simulink model "FutureGridSLs"  (R2024a)
settings: Solver=VariableStepAuto  StartTime=0.0  StopTime=600  FixedStep=1e-3  RelTol=1e-3
values from neighbouring files (symbols this model uses):
  AGG_SOL_R = inf    [FUtureGridSL.m]
  AGG_SOL_S_nom = 980e6    (= 980000000)    [FUtureGridSL.m]
  AGG_SOL_T_INV = 0.02    [FUtureGridSL.m]
  AMB_T_INV = 0.05    [FUtureGridSL.m]
  AMB_Unit_S_nom = 3e6    (= 3000000)    [FUtureGridSL.m]
  BAR_R = 0.04    [FUtureGridSL.m]
  BAR_T_ACT = 0.1    [FUtureGridSL.m]
  BAR_Unit_S_nom = 15e6    (= 15000000)    [FUtureGridSL.m]
  BRO_R_P = 0.05    [FUtureGridSL.m]    (also in Sri_Lanka_FINAL.m)
  BRO_R_T = 0.38    [FUtureGridSL.m]    (also in Sri_Lanka_FINAL.m)
  BRO_T_G = 0.2    [FUtureGridSL.m]    (also in Sri_Lanka_FINAL.m)
  BRO_T_R = 5.0    (= 5)    [FUtureGridSL.m]    (also in Sri_Lanka_FINAL.m)
  BRO_T_W = 1.0    (= 1)    [FUtureGridSL.m]    (also in Sri_Lanka_FINAL.m)
  BRO_Unit_S_nom = 17.5e6    (= 17500000)    [FUtureGridSL.m]    (also in Sri_Lanka_FINAL.m)
  BWT_R_P = 0.05    [FUtureGridSL.m]    (also in Sri_Lanka.m; Sri_Lanka_FINAL.m)
  BWT_R_T = 0.38    [FUtureGridSL.m]    (also in Sri_Lanka.m; Sri_Lanka_FINAL.m)
  BWT_T_R = 5.0    (= 5)    [FUtureGridSL.m]    (also in Sri_Lanka.m; Sri_Lanka_FINAL.m)
  BWT_T_W = 1.5    [FUtureGridSL.m]    (also in Sri_Lanka.m; Sri_Lanka_FINAL.m)
  BWT_Unit_S_nom = 40e6    (= 40000000)    [FUtureGridSL.m]    (also in Sri_Lanka.m; Sri_Lanka_FINAL.m)
  CAN_R_P = 0.05    [FUtureGridSL.m]    (also in Sri_Lanka_FINAL.m)
  CAN_R_T = 0.38    [FUtureGridSL.m]    (also in Sri_Lanka_FINAL.m)
  CAN_T_G = 0.2    [FUtureGridSL.m]    (also in Sri_Lanka_FINAL.m)
  CAN_T_R = 5.0    (= 5)    [FUtureGridSL.m]    (also in Sri_Lanka_FINAL.m)
  CAN_T_W = 1.0    (= 1)    [FUtureGridSL.m]    (also in Sri_Lanka_FINAL.m)
  CAN_Unit_S_nom = 30e6    (= 30000000)    [FUtureGridSL.m]    (also in Sri_Lanka_FINAL.m)
  D_T = 1500e6/S_base_sys    (= 1.5)    [FUtureGridSL.m]    (also in Sri_Lanka.m; Sri_Lanka_FINAL.m)
  f_base = 50    [FUtureGridSL.m]    (also in Sri_Lanka.m; Sri_Lanka_FINAL.m)
  H_eq = sum(Plant_H .* Plant_S_nom .* Plant_Status) / S_base_sys    [FUtureGridSL.m]    (also in Sri_Lanka.m = sum(Plant_H .* Plant_S_nom) / S_base_sys; Sri_Lanka_FINAL.m = sum(Plant_H .* Plant_S_nom) / S_base_sys)
  HBT_S_nom = 1.2e6    (= 1200000)    [FUtureGridSL.m]
  HBT_T_INV = 0.02    [FUtureGridSL.m]
  KEL_CC_F_GT = 0.67    [FUtureGridSL.m]    (also in Sri_Lanka.m; Sri_Lanka_FINAL.m)
  KEL_CC_F_ST = 0.33    [FUtureGridSL.m]    (also in Sri_Lanka.m; Sri_Lanka_FINAL.m)
  KEL_CC_T_HRSG = 10.0    (= 10)    [FUtureGridSL.m]    (also in Sri_Lanka.m; Sri_Lanka_FINAL.m)
  KEL_R = 0.04    [FUtureGridSL.m]    (also in Sri_Lanka.m; Sri_Lanka_FINAL.m)
  KEL_T_CH = 0.3    [FUtureGridSL.m]    (also in Sri_Lanka.m; Sri_Lanka_FINAL.m)
  KEL_UNIT1_S_nom = 20e6    (= 20000000)    [FUtureGridSL.m]    (also in Sri_Lanka.m; Sri_Lanka_FINAL.m)
  KEL_UNIT2_S_nom = 115e6    (= 115000000)    [FUtureGridSL.m]    (also in Sri_Lanka.m; Sri_Lanka_FINAL.m)
  KEL_UNIT3_S_nom = 165e6    (= 165000000)    [FUtureGridSL.m]    (also in Sri_Lanka.m; Sri_Lanka_FINAL.m)
  KOT_R_P = 0.05    [FUtureGridSL.m]
  KOT_R_T = 0.38    [FUtureGridSL.m]
  KOT_T_R = 5.0    (= 5)    [FUtureGridSL.m]
  KOT_T_W = 1.1    [FUtureGridSL.m]
  KOT_Unit_S_nom = 67e6    (= 67000000)    [FUtureGridSL.m]
  KUK_R_P = 0.05    [FUtureGridSL.m]    (also in Sri_Lanka_FINAL.m)
  KUK_R_T = 0.38    [FUtureGridSL.m]    (also in Sri_Lanka_FINAL.m)
  KUK_T_R = 5.0    (= 5)    [FUtureGridSL.m]    (also in Sri_Lanka_FINAL.m)
  KUK_T_W = 0.8    [FUtureGridSL.m]    (also in Sri_Lanka_FINAL.m)
  KUK_Unit_S_nom = 40e6    (= 40000000)    [FUtureGridSL.m]    (also in Sri_Lanka_FINAL.m)
  LAK_R = 0.04    [FUtureGridSL.m]    (also in Sri_Lanka.m; Sri_Lanka_FINAL.m)
  LAK_S_nom = 300e6    (= 300000000)    [FUtureGridSL.m]    (also in Sri_Lanka.m; Sri_Lanka_FINAL.m)
  LAU_T_INV = 0.02    [FUtureGridSL.m]
  LAU_Unit_S_nom = 20e6    (= 20000000)    [FUtureGridSL.m]
  Load_pu = 2388.8 / 1000    (= 2.3888)    [FUtureGridSL.m]
  MAD_T_INV = 0.02    [FUtureGridSL.m]
  MAD_Unit_S_nom = 100e6    (= 100000000)    [FUtureGridSL.m]
  MADK_Unit_S_nom = 12e6    (= 12000000)    [FUtureGridSL.m]
  MADU_T_INV = 0.05    [FUtureGridSL.m]
  MAM1_T_INV = 0.05    [FUtureGridSL.m]
  MAM1_Unit_S_nom = 10e6    (= 10000000)    [FUtureGridSL.m]
  MAM2_T_INV = 0.05    [FUtureGridSL.m]
  MAM2_Unit_S_nom = 10e6    (= 10000000)    [FUtureGridSL.m]
  MAM3_T_INV = 0.05    [FUtureGridSL.m]
  MAM3_Unit_S_nom = 10e6    (= 10000000)    [FUtureGridSL.m]
  MAN_T_INV = 0.05    [FUtureGridSL.m]    (also in Sri_Lanka_FINAL.m)
  MAN_Unit_S_nom = 100e6    (= 100000000)    [FUtureGridSL.m]    (also in Sri_Lanka_FINAL.m)
  NAL_T_INV = 0.05    [FUtureGridSL.m]
  NAL_Unit_S_nom = 4.8e6    (= 4800000)    [FUtureGridSL.m]
  NIR_T_INV = 0.05    [FUtureGridSL.m]
  NIR_Unit_S_nom = 10.5e6    (= 10500000)    [FUtureGridSL.m]
  NLX_R_P = 0.05    [FUtureGridSL.m]    (also in Sri_Lanka_FINAL.m)
  NLX_R_T = 0.40    (= 0.4)    [FUtureGridSL.m]    (also in Sri_Lanka_FINAL.m)
  NLX_T_G = 0.2    [FUtureGridSL.m]    (also in Sri_Lanka_FINAL.m)
  NLX_T_R = 5.0    (= 5)    [FUtureGridSL.m]    (also in Sri_Lanka_FINAL.m)
  NLX_T_W = 1.2    [FUtureGridSL.m]    (also in Sri_Lanka_FINAL.m)
  NLX_Unit_S_nom = 50e6    (= 50000000)    [FUtureGridSL.m]    (also in Sri_Lanka_FINAL.m)
  OLX_R_P = 0.05    [FUtureGridSL.m]    (also in Sri_Lanka_FINAL.m)
  OLX_R_T = 0.38    [FUtureGridSL.m]    (also in Sri_Lanka_FINAL.m)
  OLX_T_G = 0.2    [FUtureGridSL.m]    (also in Sri_Lanka_FINAL.m)
  OLX_T_R = 5.0    (= 5)    [FUtureGridSL.m]    (also in Sri_Lanka_FINAL.m)
  OLX_T_W = 1.0    (= 1)    [FUtureGridSL.m]    (also in Sri_Lanka_FINAL.m)
  OLX_Unit_S_nom_1 = 12.5e6    (= 12500000)    [FUtureGridSL.m]    (also in Sri_Lanka_FINAL.m)
  OLX_Unit_S_nom_2 = 8.33e6    (= 8330000)    [FUtureGridSL.m]    (also in Sri_Lanka_FINAL.m)
  POL_R_P = 0.05    [FUtureGridSL.m]    (also in Sri_Lanka_FINAL.m)
  POL_R_T = 0.40    (= 0.4)    [FUtureGridSL.m]    (also in Sri_Lanka_FINAL.m)
  POL_T_G = 0.2    [FUtureGridSL.m]    (also in Sri_Lanka_FINAL.m)
  POL_T_R = 5.0    (= 5)    [FUtureGridSL.m]    (also in Sri_Lanka_FINAL.m)
  POL_T_W = 1.4    [FUtureGridSL.m]    (also in Sri_Lanka_FINAL.m)
  POL_Unit_S_nom = 45e6    (= 45000000)    [FUtureGridSL.m]    (also in Sri_Lanka_FINAL.m)
  POLW_T_INV = 0.05    [FUtureGridSL.m]
  POLW_Unit_S_nom = 12e6    (= 12000000)    [FUtureGridSL.m]
  Pref_Set_AGG_SOL = (Load_pu * K_AGG_SOL)  * (S_base_sys / AGG_SOL_S_nom)    (= 0)    [FUtureGridSL.m]
  Pref_Set_AMB = (Load_pu * K_AMB) * (S_base_sys / AMB_Unit_S_nom)    (= 0)    [FUtureGridSL.m]
  Pref_Set_BAR = (Load_pu * K_BAR) * (S_base_sys / (4 * BAR_Unit_S_nom))    (= 3.98133333333)    [FUtureGridSL.m]
  Pref_Set_BRO = (Load_pu * K_BRO) * (S_base_sys / (2 * BRO_Unit_S_nom))    (= 0)    [FUtureGridSL.m]
  Pref_Set_BWT = (Load_pu * K_BWT) * (S_base_sys / (1 * BWT_Unit_S_nom))    (= 0)    [FUtureGridSL.m]
  Pref_Set_CAN = (Load_pu * K_CAN) * (S_base_sys / (2 * CAN_Unit_S_nom))    (= 0)    [FUtureGridSL.m]
  Pref_Set_HBT = (Load_pu * K_HBT)  * (S_base_sys / HBT_S_nom)    (= 0)    [FUtureGridSL.m]
  Pref_Set_KEL1 = (Load_pu * K_KEL1)  * (S_base_sys / (4*KEL_UNIT1_S_nom))    (= 0)    [FUtureGridSL.m]
  Pref_Set_KEL2 = (Load_pu * K_KEL2)  * (S_base_sys / (KEL_UNIT2_S_nom ))    (= 0)    [FUtureGridSL.m]
  Pref_Set_KEL3 = (Load_pu * K_KEL3)  * (S_base_sys / (KEL_UNIT3_S_nom))    (= 0)    [FUtureGridSL.m]
  Pref_Set_KOT = (Load_pu * K_KOT)  * (S_base_sys / (3 * KOT_Unit_S_nom))    (= 0.986419900498)    [FUtureGridSL.m]
  Pref_Set_KUK = (Load_pu * K_KUK) * (S_base_sys / (2 * KUK_Unit_S_nom))    (= 0)    [FUtureGridSL.m]
  Pref_Set_LAK = (Load_pu * K_LAK)  * (S_base_sys / (3 * LAK_S_nom))    (= 0.177302044444)    [FUtureGridSL.m]
  Pref_Set_LAU = (Load_pu * K_LAU)  * (S_base_sys / LAU_Unit_S_nom)    (= 1.1944)    [FUtureGridSL.m]
  Pref_Set_MAD = (Load_pu * K_MAD)  * (S_base_sys / MAD_Unit_S_nom)    (= 0.7333616)    [FUtureGridSL.m]
  Pref_Set_MADK = (Load_pu * K_MADK) * (S_base_sys / AMB_Unit_S_nom)    (= 0)    [FUtureGridSL.m]
  Pref_Set_MAM1 = (Load_pu * K_MAM1) * (S_base_sys / MAM1_Unit_S_nom)    (= 0)    [FUtureGridSL.m]
  Pref_Set_MAM2 = (Load_pu * K_MAM2) * (S_base_sys / MAM2_Unit_S_nom)    (= 0)    [FUtureGridSL.m]
  Pref_Set_MAM3 = (Load_pu * K_MAM3) * (S_base_sys / MAM3_Unit_S_nom)    (= 0)    [FUtureGridSL.m]
  Pref_Set_MAN = (Load_pu * K_MAN)  * (S_base_sys / MAN_Unit_S_nom)    (= 0.035832)    [FUtureGridSL.m]
  Pref_Set_NAL = (Load_pu * K_NAL) * (S_base_sys / NAL_Unit_S_nom)    (= 0)    [FUtureGridSL.m]
  Pref_Set_NIR = (Load_pu * K_NIR) * (S_base_sys / NIR_Unit_S_nom)    (= 0)    [FUtureGridSL.m]
  Pref_Set_NLX = (Load_pu * K_NLX)  * (S_base_sys / (2 * NLX_Unit_S_nom))    (= 0)    [FUtureGridSL.m]
  Pref_Set_OLX1 = (Load_pu * K_OLX1) * (S_base_sys / (2 * OLX_Unit_S_nom_1))    (= 0)    [FUtureGridSL.m]
  Pref_Set_OLX2 = (Load_pu * K_OLX2) * (S_base_sys / (3 * OLX_Unit_S_nom_2))    (= 0)    [FUtureGridSL.m]
  Pref_Set_POL = (Load_pu * K_POL) * (S_base_sys / (2 * POL_Unit_S_nom))    (= 0)    [FUtureGridSL.m]
  Pref_Set_POLW = (Load_pu * K_POLW) * (S_base_sys / POLW_Unit_S_nom)    (= 0)    [FUtureGridSL.m]
  Pref_Set_PWD = (Load_pu * K_PWD) * (S_base_sys / PWD_Unit_S_nom)    (= 0)    [FUtureGridSL.m]
  Pref_Set_RAN = (Load_pu * K_RAN) * (S_base_sys / (2 * RAN_Unit_S_nom))    (= 9.47936507937)    [FUtureGridSL.m]
  Pref_Set_RTB = (Load_pu * K_RTB) * (S_base_sys / (2 * RTB_Unit_S_nom))    (= 0)    [FUtureGridSL.m]
  ... (+116 more)
(part 2 of 2)

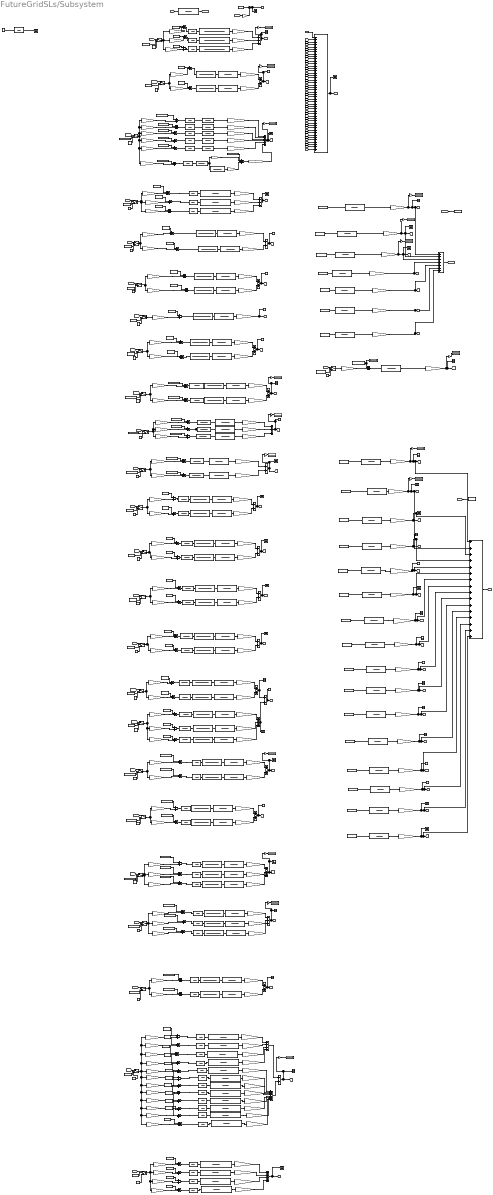
== system FutureGridSLs/Subsystem ==
  note: HambanthotaSolarFarm
  note: [Steam Turbine Path: 33%]
  note: [Gas Turbine Path: 67%]
  note: SAMANALAWEWA
  note: GRID BLOCK
  note: SUMMING BLOCK
  note: To convert to the frequency
  note: LAKVIJAYA
  note: KELANITISSA
  note: Uthuru Janani plant
  note: RANDENIGALA
  note: RANTAMBE
  note: BOWATENNA
  note: UKUWELA
  note: Yugadhanavi GT and ST
  note: New LAXAPANA
  note: Sobadhanavi ST and GT
  note: Polpitiya Plant
  note: Canyon Plant
  note: Wimalasurendra Plant
  note: Kukuleganga Plant
  note: Uma Oya Plant
  note: Old Laxapana Plant
  note: Broadland Plant
  note: Victoria Plant
  note: Upper Kotmale Plant
  note: Kotmale Plant
  note: Colombo Port Barge Plant
  note: Sapugaskanda Plant
  note: Uppudaluwa Wind Farm
  note: Maduru Oya Solar PV subsystem
  note: LAUGFS Hambantota Solar Power Plant
  note: Solar One Ceylon Solar Farm
  note: THAMBAPAVANI WIND FARM: 100 MW
  note: SagaSolarFarm
  note: Suryashakthi 1 SolarFarm
  note: Suryashakthi 2 SolarFarm
  note: Ambewela Aitken Spence Wind Farm
  note: Madurankuliya Wind Farm
  note: Mampuri I Wind Farm
  note: Mampuri II Wind Farm
  note: Mampuri III Wind Farm
  note: Nala Danavi Wind Farm
  note: Nirmalapura Wind Farm
  note: Pawan Danavi Wind Farm
  note: Pollupalai Wind Farm
  note: Seguwantivu Wind Farm
  note: Vallimunai Wind Farm
  note: Vidatamunai Wind Farm
  note: Willwind Wind Farm
  note: Wind scape Farm
  note: Forecasted Solar PV Farm (IBR)
  Load Disturbance : Inport
  " " : TransferFcn  Denominator=[2*H_eq D_T]
  Actuator Delay : TransferFcn  Denominator="[UTH_T_ACT  1]"
  Actuator Delay1 : TransferFcn  Denominator="[UTH_T_ACT  1]"
  Actuator Delay{3..13,15} (12 alike) : TransferFcn  Denominator="[SAP_T_ACT  1]"
  Actuator Delay{14,16..18} (4 alike) : TransferFcn  Denominator="[BAR_T_ACT  1]"
  Actuator Delay2 : TransferFcn  Denominator="[UTH_T_ACT  1]"
  Add{,4,8,13,20..21} (6 alike) : Sum  Inputs=+++
  Add1 : Sum  Inputs=-+++++++++++++++++++++++++++++++++++++++++++++++
  Add{2,5..7,9..12,14..19,22,25,27,29..65,67..98} (86 alike) : Sum
  Add23 : Sum  Inputs=++++
  Add24 : Sum  Inputs=++++++++
  Add26 : Sum  Inputs=++++
  Add28 : Sum  Inputs=+++++++
  Add3 : Sum  Inputs=++++++
  Add66 : Sum  Inputs=++++++++++++++++
  Base Scaling Gain : Gain  Gain=SAM_Unit_S_nom / S_base_sys
  Base Scaling Gain GT : Gain  Gain=YUGA_GT_S_nom / S_base_sys
  Base Scaling Gain GT1 : Gain  Gain=YUGA_GT_S_nom / S_base_sys
  Base Scaling Gain GT2 : Gain  Gain=SOBA_GT_S_nom / S_base_sys
  Base Scaling Gain1 : Gain  Gain=SAM_Unit_S_nom / S_base_sys
  Base Scaling Gain10 : Gain  Gain=RTB_Unit_S_nom / S_base_sys
  Base Scaling Gain11 : Gain  Gain=UKU_Unit_S_nom / S_base_sys
  Base Scaling Gain12 : Gain  Gain=BWT_Unit_S_nom / S_base_sys
  Base Scaling Gain13 : Gain  Gain=UKU_Unit_S_nom / S_base_sys
  Base Scaling Gain14 : Gain  Gain=MAN_Unit_S_nom / S_base_sys
  Base Scaling Gain15 : Gain  Gain=SOBA_ST_S_nom/S_base_sys
  Base Scaling Gain16 : Gain  Gain=YUGA_ST_S_nom/S_base_sys
  Base Scaling Gain17 : Gain  Gain=NLX_Unit_S_nom / S_base_sys
  Base Scaling Gain18 : Gain  Gain=NLX_Unit_S_nom / S_base_sys
  Base Scaling Gain19 : Gain  Gain=POL_Unit_S_nom / S_base_sys
  Base Scaling Gain2 : Gain  Gain=RTB_Unit_S_nom / S_base_sys
  Base Scaling Gain20 : Gain  Gain=POL_Unit_S_nom / S_base_sys
  Base Scaling Gain21 : Gain  Gain=WIM_Unit_S_nom / S_base_sys
  Base Scaling Gain22 : Gain  Gain=WIM_Unit_S_nom / S_base_sys
  Base Scaling Gain23 : Gain  Gain=BRO_Unit_S_nom / S_base_sys
  Base Scaling Gain24 : Gain  Gain=BRO_Unit_S_nom / S_base_sys
  Base Scaling Gain25 : Gain  Gain=OLX_Unit_S_nom_1 / S_base_sys
  Base Scaling Gain26 : Gain  Gain=OLX_Unit_S_nom_1 / S_base_sys
  Base Scaling Gain27 : Gain  Gain=OLX_Unit_S_nom_2 / S_base_sys
  Base Scaling Gain28 : Gain  Gain=OLX_Unit_S_nom_2 / S_base_sys
  Base Scaling Gain29 : Gain  Gain=OLX_Unit_S_nom_2 / S_base_sys
  Base Scaling Gain{3..6} (4 alike) : Gain  Gain=KEL_UNIT1_S_nom/ S_base_sys
  Base Scaling Gain30 : Gain  Gain=UMA_Unit_S_nom / S_base_sys
  Base Scaling Gain31 : Gain  Gain=UMA_Unit_S_nom / S_base_sys
  Base Scaling Gain32 : Gain  Gain=KUK_Unit_S_nom / S_base_sys
  Base Scaling Gain33 : Gain  Gain=KUK_Unit_S_nom / S_base_sys
  Base Scaling Gain34 : Gain  Gain=CAN_Unit_S_nom / S_base_sys
  Base Scaling Gain35 : Gain  Gain=CAN_Unit_S_nom / S_base_sys
  Base Scaling Gain36 : Gain  Gain=VIC_Unit_S_nom / S_base_sys
  Base Scaling Gain37 : Gain  Gain=VIC_Unit_S_nom / S_base_sys
  Base Scaling Gain38 : Gain  Gain=VIC_Unit_S_nom / S_base_sys
  Base Scaling Gain39 : Gain  Gain=KOT_Unit_S_nom / S_base_sys
  Base Scaling Gain40 : Gain  Gain=KOT_Unit_S_nom / S_base_sys
  Base Scaling Gain41 : Gain  Gain=UKT_Unit_S_nom / S_base_sys
  Base Scaling Gain42 : Gain  Gain=UKT_Unit_S_nom / S_base_sys
  Base Scaling Gain43 : Gain  Gain=KOT_Unit_S_nom / S_base_sys
  Base Scaling Gain44 : Gain  Gain=MAD_Unit_S_nom / S_base_sys
  Base Scaling Gain45 : Gain  Gain=LAU_Unit_S_nom / S_base_sys
  Base Scaling Gain46 : Gain  Gain=SOC_S_nom / S_base_sys
  Base Scaling Gain47 : Gain  Gain=UPP_Unit_S_nom / S_base_sys
  Base Scaling Gain49 : Gain  Gain=HBT_S_nom / S_base_sys
  Base Scaling Gain50 : Gain  Gain=SAG_S_nom / S_base_sys
  Base Scaling Gain51 : Gain  Gain=SS1_S_nom / S_base_sys
  Base Scaling Gain52 : Gain  Gain=SS2_S_nom / S_base_sys
  Base Scaling Gain53 : Gain  Gain=AMB_Unit_S_nom / S_base_sys
  Base Scaling Gain54 : Gain  Gain=MADK_Unit_S_nom / S_base_sys
  Base Scaling Gain55 : Gain  Gain=MAM1_Unit_S_nom / S_base_sys
  Base Scaling Gain56 : Gain  Gain=MAM2_Unit_S_nom / S_base_sys
  Base Scaling Gain57 : Gain  Gain=MAM3_Unit_S_nom / S_base_sys
  Base Scaling Gain58 : Gain  Gain=NAL_Unit_S_nom / S_base_sys
  Base Scaling Gain59 : Gain  Gain=NIR_Unit_S_nom / S_base_sys
  Base Scaling Gain60 : Gain  Gain=PWD_Unit_S_nom / S_base_sys
  Base Scaling Gain61 : Gain  Gain=POLW_Unit_S_nom / S_base_sys
  Base Scaling Gain62 : Gain  Gain=SEG_Unit_S_nom / S_base_sys
  Base Scaling Gain63 : Gain  Gain=AGG_SOL_S_nom / S_base_sys
  Base Scaling Gain64 : Gain  Gain=VALL_Unit_S_nom / S_base_sys
  Base Scaling Gain65 : Gain  Gain=VID_Unit_S_nom / S_base_sys
  Base Scaling Gain66 : Gain  Gain=WILL_Unit_S_nom / S_base_sys
  Base Scaling Gain67 : Gain  Gain=WSC_Unit_S_nom / S_base_sys
  Base Scaling Gain7 : Gain  Gain=KEL_UNIT2_S_nom/ S_base_sys
  Base Scaling Gain8 : Gain  Gain=RAN_Unit_S_nom / S_base_sys
  Base Scaling Gain9 : Gain  Gain=RAN_Unit_S_nom / S_base_sys
  Combustr : TransferFcn  Denominator="[KEL_T_CH  1]"
  Constant : Constant  Value=f_base
  Constant{1,15..16,143} (4 alike) : Constant  Value=Pref_Set_LAK
  Constant10 : Constant  Value=Pref_Set_MAN
  Constant{22,96..118,127,144} (26 alike) : Constant  Value=0
  Constant11 : Constant  Value=Pref_Set_MAD
  Constant{92..95,119} (5 alike) : Constant  Value=Pref_Set_BAR
  Constant12 : Constant  Value=Pref_Set_LAU
  Constant{33..36,120} (5 alike) : Constant  Value=Pref_Set_SAP_A
  Constant121 : Constant  Value=Pref_Set_UKT
  Constant{30..32,122} (4 alike) : Constant  Value=Pref_Set_KOT
  Constant{27..29,123} (4 alike) : Constant  Value=Pref_Set_VIC
  Constant124 : Constant  Value=Pref_Set_KUK
  Constant125 : Constant  Value=Pref_Set_UMA
  Constant126 : Constant  Value=Pref_Set_OLX1
  Constant{85..87,128} (4 alike) : Constant  Value=Pref_Set_OLX2
  Constant129 : Constant  Value=Pref_Set_BRO
  Constant13 : Constant  Value=Pref_Set_SOC
  Constant130 : Constant  Value=Pref_Set_WIM
  Constant131 : Constant  Value=Pref_Set_CAN
  Constant132 : Constant  Value=Pref_Set_POL
  Constant133 : Constant  Value=Pref_Set_SOBA1
  Constant134 : Constant  Value=Pref_Set_YUGA1
  Constant135 : Constant  Value=Pref_Set_NLX
  Constant136 : Constant  Value=Pref_Set_UKU
  Constant137 : Constant  Value=Pref_Set_BWT
  Constant138 : Constant  Value=Pref_Set_RTB
  Constant139 : Constant  Value=Pref_Set_RAN
  Constant14 : Constant  Value=Pref_Set_UPP
  Constant{61,66..67,140} (4 alike) : Constant  Value=Pref_Set_UTH
  Constant{5,18..20,141} (5 alike) : Constant  Value=Pref_Set_KEL1
  Constant142 : Constant  Value=Pref_Set_SAM
  Constant145 : Constant  Value=Pref_Set_AGG_SOL
  Constant146 : Constant  Value=Pref_Set_AGG_SOL
  Constant17 : Constant  Value=Pref_Set_SAM
  Constant2 : Constant
  Constant21 : Constant  Value=Pref_Set_KEL2
  Constant23 : Constant  Value=Pref_Set_NLX
  Constant24 : Constant  Value=Pref_Set_NLX
  Constant25 : Constant  Value=Pref_Set_UMA
  Constant26 : Constant  Value=Pref_Set_UMA
  Constant{37..44} (8 alike) : Constant  Value=Pref_Set_SAP_B
  Constant4 : Constant  Value=Pref_Set_SAM
  Constant45 : Constant  Value=Pref_Set_SOBA1
  Constant46 : Constant  Value=Pref_Set_SOBA2
  Constant47 : Constant  Value=Pref_Set_HBT
  Constant48 : Constant  Value=Pref_Set_SAG
  Constant49 : Constant  Value=Pref_Set_SS1
  Constant50 : Constant  Value=Pref_Set_SS2
  Constant51 : Constant  Value=Pref_Set_AMB
  Constant52 : Constant  Value=Pref_Set_MADK
  Constant53 : Constant  Value=Pref_Set_MAM1
  Constant54 : Constant  Value=Pref_Set_MAM2
  Constant55 : Constant  Value=Pref_Set_MAM3
  Constant56 : Constant  Value=Pref_Set_NAL
  Constant57 : Constant  Value=Pref_Set_NIR
  Constant58 : Constant  Value=Pref_Set_PWD
  Constant59 : Constant  Value=Pref_Set_POLW
  Constant6 : Constant  Value=Pref_Set_YUGA1
  Constant60 : Constant  Value=Pref_Set_SEG
  Constant62 : Constant  Value=Pref_Set_VALL
  Constant63 : Constant  Value=Pref_Set_VID
  Constant64 : Constant  Value=Pref_Set_WILL
  Constant65 : Constant  Value=Pref_Set_WSC
  Constant68 : Constant  Value=Pref_Set_RAN
  Constant69 : Constant  Value=Pref_Set_RAN
  Constant7 : Constant  Value=Pref_Set_YUGA1
  Constant70 : Constant  Value=Pref_Set_RTB
  Constant71 : Constant  Value=Pref_Set_RTB
  Constant72 : Constant  Value=Pref_Set_BWT
  Constant73 : Constant  Value=Pref_Set_UKU
  Constant74 : Constant  Value=Pref_Set_UKU
  Constant75 : Constant  Value=Pref_Set_POL
  Constant76 : Constant  Value=Pref_Set_POL
  Constant77 : Constant  Value=Pref_Set_CAN
  Constant78 : Constant  Value=Pref_Set_CAN
  Constant79 : Constant  Value=Pref_Set_WIM
  Constant8 : Constant  Value=Pref_Set_YUGA2
  Constant80 : Constant  Value=Pref_Set_WIM
  Constant81 : Constant  Value=Pref_Set_BRO
  Constant82 : Constant  Value=Pref_Set_BRO
  Constant83 : Constant  Value=Pref_Set_OLX1
  Constant84 : Constant  Value=Pref_Set_OLX1
  Constant88 : Constant  Value=Pref_Set_KUK
  Constant89 : Constant  Value=Pref_Set_KUK
  Constant9 : Constant  Value=Pref_Set_KEL3
  Constant90 : Constant  Value=Pref_Set_UKT
  Constant91 : Constant  Value=Pref_Set_UKT
  Display{,1..16} (17 alike) : Display
  Gain{,4..8,13..18} (12 alike) : Gain  Gain=1e3
  Gain1 : Gain  Gain=KEL_CC_F_ST
  Gain10 : Gain  Gain=(3*VIC_Unit_S_nom)/ 1e6
  Gain11 : Gain  Gain=(3*KOT_Unit_S_nom)/ 1e6
  Gain12 : Gain  Gain=(4*SAP_A_Unit_S_nom + 8*SAP_B_Unit_S_nom)/1e6
  Gain2 : Gain  Gain=KEL_UNIT3_S_nom/ S_base_sys
  Gain3 : Gain  Gain=f_base
  Gain9 : Gain  Gain=(2*UMA_Unit_S_nom)/ 1e6
  Governer{,1..13} (14 alike) : TransferFcn  Denominator=[T_G 1]
  Governer {1..2,7,9,11,13,15,17..19,30..33,35..46} (26 alike) : TransferFcn  Denominator=[T_G 1]
  Governer {8,10,12,14,16} (5 alike) : TransferFcn  Denominator="[KEL_T_CH  1]"
  Governer 20 : TransferFcn  Denominator=[CAN_T_G 1]
  Governer 21 : TransferFcn  Denominator="[WIM_T_G  1]"
  Governer 22 : TransferFcn  Denominator="[WIM_T_G  1]"
  Governer 23 : TransferFcn  Denominator="[BRO_T_G  1]"
  Governer 24 : TransferFcn  Denominator="[BRO_T_G  1]"
  Governer {25..29} (5 alike) : TransferFcn  Denominator="[OLX_T_G  1]"
  Governer 3 : TransferFcn  Denominator=[POL_T_G 1]
  Governer 34 : TransferFcn  Denominator="[CAN_T_G  1]"
  Governer 4 : TransferFcn  Denominator=[POL_T_G 1]
  Governer 47 : TransferFcn  Denominator=[100 1]
  Governer 5 : TransferFcn  Denominator=[NLX_T_G 1]
  Governer 6 : TransferFcn  Denominator=[NLX_T_G 1]
  Governer GT : TransferFcn  Denominator=[YUGA_GT_T_G 1]
  Governer GT1 : TransferFcn  Denominator=[YUGA_GT_T_G 1]
  Governer GT2 : TransferFcn  Denominator=[SOBA_GT_T_g 1]
  Governer ST : TransferFcn  Denominator=[YUGA_ST_T_ch 1]
  Governer ST1 : TransferFcn  Denominator=[SOBA_ST_T_ch 1]
  HRSG Delay : TransferFcn  Denominator="[KEL_CC_T_HRSG  1]"
  Inverter Delay : TransferFcn  Denominator="[MAN_T_INV  1]"
  Inverter Delay1 : TransferFcn  Denominator=[MAD_T_INV 1]
  Inverter Delay10 : TransferFcn  Denominator=[MADU_T_INV 1]
  Inverter Delay11 : TransferFcn  Denominator=[MAM1_T_INV 1]
  Inverter Delay12 : TransferFcn  Denominator=[MAM2_T_INV 1]
  Inverter Delay13 : TransferFcn  Denominator=[MAM3_T_INV 1]
  Inverter Delay14 : TransferFcn  Denominator=[NAL_T_INV 1]
  Inverter Delay15 : TransferFcn  Denominator=[NIR_T_INV 1]
  Inverter Delay16 : TransferFcn  Denominator=[PWD_T_INV 1]
  Inverter Delay17 : TransferFcn  Denominator=[POLW_T_INV 1]
  Inverter Delay18 : TransferFcn  Denominator=[SEG_T_INV 1]
  Inverter Delay2 : TransferFcn  Denominator=[LAU_T_INV 1]
  Inverter Delay20 : TransferFcn  Denominator=[VALL_T_INV 1]
  Inverter Delay21 : TransferFcn  Denominator=[VID_T_INV 1]
  Inverter Delay22 : TransferFcn  Denominator=[WILL_T_INV 1]
  Inverter Delay23 : TransferFcn  Denominator=[WSC_T_INV 1]
  Inverter Delay3 : TransferFcn  Denominator=[SOC_T_INV 1]
  Inverter Delay4 : TransferFcn  Denominator=[UPP_T_INV 1]
  Inverter Delay5 : TransferFcn  Denominator=[HBT_T_INV 1]
  Inverter Delay6 : TransferFcn  Denominator=[SAG_T_INV 1]
  Inverter Delay7 : TransferFcn  Denominator=[SS1_T_INV 1]
  Inverter Delay8 : TransferFcn  Denominator=[SS2_T_INV 1]
  Inverter Delay9 : TransferFcn  Denominator=[AMB_T_INV 1]
  PURE DROOP : Gain  Gain=-1/LAK_R
  PURE DROOP GT : Gain  Gain=-1/YUGA_GT_R
  PURE DROOP GT1 : Gain  Gain=-1/YUGA_GT_R
  PURE DROOP GT2 : Gain  Gain=-1/SOBA_GT_R
  PURE DROOP ST : Gain  Gain=-1/YUGA_ST_R
  PURE DROOP ST1 : Gain  Gain=-1/SOBA_ST_R
  PURE DROOP1 : Gain  Gain=-1/LAK_R
  PURE DROOP{6..11} (6 alike) : Gain  Gain=-1/KEL_R
  PURE DROOP12 : Gain  Gain=-1/UTH_R
  PURE DROOP13 : Gain  Gain=-1/UTH_R
  PURE DROOP14 : Gain  Gain=-1/UTH_R
  PURE DROOP15 : Gain  Gain=-1/RAN_R_P
  PURE DROOP16 : Gain  Gain=-1/RAN_R_P
  PURE DROOP17 : Gain  Gain=-1/RTB_R_P
  PURE DROOP18 : Gain  Gain=-1/UKU_R_P
  PURE DROOP19 : Gain  Gain=-1/BWT_R_P
  PURE DROOP2 : Gain  Gain=-1/LAK_R
  PURE DROOP20 : Gain  Gain=-1/UKU_R_P
  PURE DROOP21 : Gain  Gain=-1/AGG_SOL_R
  PURE DROOP22 : Gain  Gain=-1/NLX_R_P
  PURE DROOP23 : Gain  Gain=-1/NLX_R_P
  PURE DROOP24 : Gain  Gain=-1/POL_R_P
  PURE DROOP25 : Gain  Gain=-1/POL_R_P
  PURE DROOP26 : Gain  Gain=-1/CAN_R_P
  PURE DROOP27 : Gain  Gain=-1/WIM_R_P
  PURE DROOP28 : Gain  Gain=-1/WIM_R_P
  PURE DROOP29 : Gain  Gain=-1/BRO_R_P
  PURE DROOP3 : Gain  Gain=-1/SAM_R_P
  PURE DROOP30 : Gain  Gain=-1/BRO_R_P
  PURE DROOP{31..35} (5 alike) : Gain  Gain=-1/OLX_R_P
  PURE DROOP36 : Gain  Gain=-1/UMA_R_P
  PURE DROOP37 : Gain  Gain=-1/UMA_R_P
  PURE DROOP38 : Gain  Gain=-1/KUK_R_P
  PURE DROOP39 : Gain  Gain=-1/KUK_R_P
  PURE DROOP4 : Gain  Gain=-1/SAM_R_P
  PURE DROOP40 : Gain  Gain=-1/CAN_R_P
  PURE DROOP41 : Gain  Gain=-1/VIC_R_P
  PURE DROOP42 : Gain  Gain=-1/VIC_R_P
  PURE DROOP43 : Gain  Gain=-1/VIC_R_P
  PURE DROOP44 : Gain  Gain=-1/KOT_R_P
  PURE DROOP45 : Gain  Gain=-1/KOT_R_P
  PURE DROOP46 : Gain  Gain=-1/UKT_R_P
  PURE DROOP47 : Gain  Gain=-1/UKT_R_P
  PURE DROOP48 : Gain  Gain=-1/KOT_R_P
  PURE DROOP{49..60} (12 alike) : Gain  Gain=-1/SAP_R
  PURE DROOP5 : Gain  Gain=-1/RTB_R_P
  PURE DROOP{61..64} (4 alike) : Gain  Gain=-1/BAR_R
  Scaling : Sum  Inputs=+++
  Scaling 1 : Gain  Gain=LAK_S_nom / S_base_sys
  Scaling {7..10} (4 alike) : Gain  Gain=SAP_A_Unit_S_nom / S_base_sys
  Scaling {11..18} (8 alike) : Gain  Gain=SAP_B_Unit_S_nom / S_base_sys
  Scaling {19..22} (4 alike) : Gain  Gain=BAR_Unit_S_nom / S_base_sys
  Scaling 2 : Gain  Gain=LAK_S_nom / S_base_sys
  Scaling 3 : Gain  Gain=LAK_S_nom / S_base_sys
  Scaling 4 : Gain  Gain=UTH_Unit_S_nom / S_base_sys
  Scaling 5 : Gain  Gain=UTH_Unit_S_nom / S_base_sys
  Scaling 6 : Gain  Gain=UTH_Unit_S_nom / S_base_sys
  Scope{,1..31,33..47} (47 alike) : Scope
  Scope32 : Scope  NumInputPorts=2
  Sum : Sum  Inputs=|++
  "Switch " : Switch  Criteria=u2 > Threshold  SaturateOnIntegerOverflow=off  InputSameDT=off
  Switch{1..24} (24 alike) : Switch  Criteria=u2 > Threshold  SaturateOnIntegerOverflow=off  InputSameDT=off
  To Workspace : ToWorkspace  VariableName=SOLAR_TOT  SaveFormat=Timeseries  SampleTime=-1
  To Workspace1 : ToWorkspace  VariableName=WIND_TOT  SaveFormat=Timeseries  SampleTime=-1
  Transient Droop : TransferFcn  Numerator="[SAM_T_R  1]"  Denominator="[SAM_T_R*(SAM_R_T/SAM_R_P)  1]"
  Transient Droop GT : TransferFcn  Denominator="[YUGA_GT_T_t  1]"
  Transient Droop GT1 : TransferFcn  Denominator="[YUGA_GT_T_t  1]"
  Transient Droop GT2 : TransferFcn  Denominator="[SOBA_GT_T_t  1]"
  Transient Droop ST : TransferFcn  Denominator="[YUGA_ST_T_hrsga  1]"
  Transient Droop ST1 : TransferFcn  Denominator="[SOBA_ST_T_hrsga  1]"
  Transient Droop1 : TransferFcn  Numerator="[SAM_T_R  1]"  Denominator="[SAM_T_R*(SAM_R_T/SAM_R_P)  1]"
  Transient Droop10 : TransferFcn  Numerator="[NLX_T_R  1]"  Denominator="[NLX_T_R*(NLX_R_T/NLX_R_P)  1]"
  Transient Droop11 : TransferFcn  Numerator=[POL_T_R 1]  Denominator="[POL_T_R*(POL_R_T/POL_R_P)  1]"
  Transient Droop12 : TransferFcn  Numerator="[POL_T_R  1]"  Denominator="[POL_T_R*(POL_R_T/POL_R_P)  1]"
  Transient Droop13 : TransferFcn  Numerator=[BRO_T_R 1]  Denominator="[BRO_T_R*(BRO_R_T/BRO_R_P)  1]"
  Transient Droop14 : TransferFcn  Numerator=[BRO_T_R 1]  Denominator="[BRO_T_R*(BRO_R_T/BRO_R_P)  1]"
  Transient Droop{15..19} (5 alike) : TransferFcn  Numerator=[OLX_T_R 1]  Denominator="[OLX_T_R*(OLX_R_T/OLX_R_P)  1]"
  Transient Droop2 : TransferFcn  Numerator="[RAN_T_R  1]"  Denominator="[(RAN_R_T / RAN_R_P) * RAN_T_R   1]"
  Transient Droop20 : TransferFcn  Numerator="[UMA_T_R  1]"  Denominator="[UMA_T_R*(UMA_R_T/UMA_R_P)  1]"
  Transient Droop21 : TransferFcn  Numerator="[UMA_T_R  1]"  Denominator="[UMA_T_R*(UMA_R_T/UMA_R_P)  1]"
  Transient Droop22 : TransferFcn  Numerator="[KUK_T_R  1]"  Denominator="[KUK_T_R*(KUK_R_T/KUK_R_P)  1]"
  Transient Droop23 : TransferFcn  Numerator="[KUK_T_R  1]"  Denominator="[KUK_T_R*(KUK_R_T/KUK_R_P)  1]"
  Transient Droop24 : TransferFcn  Numerator=[CAN_T_R 1]  Denominator="[CAN_T_R*(CAN_R_T/CAN_R_P)  1]"
  Transient Droop25 : TransferFcn  Numerator=[CAN_T_R 1]  Denominator="[CAN_T_R*(CAN_R_T/CAN_R_P)  1]"
  Transient Droop26 : TransferFcn  Numerator=[WIM_T_R 1]  Denominator="[WIM_T_R*(WIM_R_T/WIM_R_P)  1]"
  Transient Droop27 : TransferFcn  Numerator=[WIM_T_R 1]  Denominator="[WIM_T_R*(WIM_R_T/WIM_R_P)  1]"
  Transient Droop28 : TransferFcn  Numerator="[VIC_T_R  1]"  Denominator="[VIC_T_R*(VIC_R_T/VIC_R_P)  1]"
  Transient Droop29 : TransferFcn  Numerator="[VIC_T_R  1]"  Denominator="[VIC_T_R*(VIC_R_T/VIC_R_P)  1]"
  Transient Droop3 : TransferFcn  Numerator="[RAN_T_R  1]"  Denominator="[(RAN_R_T / RAN_R_P) * RAN_T_R   1]"
  Transient Droop30 : TransferFcn  Numerator="[VIC_T_R  1]"  Denominator="[VIC_T_R*(VIC_R_T/VIC_R_P)  1]"
  Transient Droop31 : TransferFcn  Numerator="[KOT_T_R  1]"  Denominator="[KOT_T_R*(KOT_R_T/KOT_R_P)  1]"
  Transient Droop32 : TransferFcn  Numerator="[KOT_T_R  1]"  Denominator="[KOT_T_R*(KOT_R_T/KOT_R_P)  1]"
  Transient Droop33 : TransferFcn  Numerator="[UKT_T_R  1]"  Denominator="[UKT_T_R*(UKT_R_T/UKT_R_P)  1]"
  Transient Droop34 : TransferFcn  Numerator="[UKT_T_R  1]"  Denominator="[UKT_T_R*(UKT_R_T/UKT_R_P)  1]"
  Transient Droop35 : TransferFcn  Numerator="[KOT_T_R  1]"  Denominator="[KOT_T_R*(KOT_R_T/KOT_R_P)  1]"
  Transient Droop37 : TransferFcn  Denominator=[AGG_SOL_T_INV, 1]
  Transient Droop4 : TransferFcn  Numerator="[RTB_T_R  1]"  Denominator="[(RTB_R_T / RTB_R_P) * RTB_T_R   1]"
  Transient Droop5 : TransferFcn  Numerator="[RTB_T_R  1]"  Denominator="[(RTB_R_T / RTB_R_P) * RTB_T_R   1]"
  Transient Droop6 : TransferFcn  Numerator="[BWT_T_R  1]"  Denominator="[(BWT_R_T / BWT_R_P) * BWT_T_R   1]"
  Transient Droop7 : TransferFcn  Numerator="[UKU_T_R  1]"  Denominator="[(UKU_R_T / UKU_R_P) * UKU_T_R   1]"
  Transient Droop8 : TransferFcn  Numerator="[UKU_T_R  1]"  Denominator="[(UKU_R_T / UKU_R_P) * UKU_T_R   1]"
  Transient Droop9 : TransferFcn  Numerator=[NLX_T_R 1]  Denominator="[NLX_T_R*(NLX_R_T/NLX_R_P)  1]"
  Turbine Dynamics (Reheat) : TransferFcn  Numerator="[RHT_F_HP*RHT_T_RH  1]"  Denominator="[RHT_T_CH*RHT_T_RH  (RHT_T_CH+RHT_T_RH)  1]"
  Turbine Dynamics (Reheat)1 : TransferFcn  Numerator="[RHT_F_HP*RHT_T_RH  1]"  Denominator="[RHT_T_CH*RHT_T_RH  (RHT_T_CH+RHT_T_RH)  1]"
  Turbine Dynamics (Reheat)2 : TransferFcn  Numerator="[RHT_F_HP*RHT_T_RH  1]"  Denominator="[RHT_T_CH*RHT_T_RH  (RHT_T_CH+RHT_T_RH)  1]"
  Water Column : TransferFcn  Numerator="[-SAM_T_W  1]"  Denominator="[0.5*SAM_T_W  1]"
  Water Column1 : TransferFcn  Numerator="[-SAM_T_W  1]"  Denominator="[0.5*SAM_T_W  1]"
  Water Column10 : TransferFcn  Numerator="[-NLX_T_W  1]"  Denominator="[0.5*NLX_T_W  1]"
  Water Column11 : TransferFcn  Numerator="[-POL_T_W  1]"  Denominator="[0.5*POL_T_W  1]"
  Water Column12 : TransferFcn  Numerator="[-POL_T_W  1]"  Denominator="[0.5*POL_T_W  1]"
  Water Column13 : TransferFcn  Numerator="[-BRO_T_W  1]"  Denominator="[0.5*BRO_T_W  1]"
  Water Column14 : TransferFcn  Numerator="[-BRO_T_W  1]"  Denominator="[0.5*BRO_T_W  1]"
  Water Column{15..19} (5 alike) : TransferFcn  Numerator="[-OLX_T_W  1]"  Denominator="[0.5*OLX_T_W  1]"
  Water Column2 : TransferFcn  Numerator="[-RAN_T_W  1]"  Denominator="[0.5 * RAN_T_W   1]"
  Water Column20 : TransferFcn  Numerator="[-UMA_T_W  1]"  Denominator="[0.5*UMA_T_W  1]"
  Water Column21 : TransferFcn  Numerator="[-UMA_T_W  1]"  Denominator="[0.5*UMA_T_W  1]"
  Water Column22 : TransferFcn  Numerator="[-KUK_T_W  1]"  Denominator="[0.5*KUK_T_W  1]"
  Water Column23 : TransferFcn  Numerator="[-KUK_T_W  1]"  Denominator="[0.5*KUK_T_W  1]"
  Water Column24 : TransferFcn  Numerator="[-CAN_T_W  1]"  Denominator="[0.5*CAN_T_W  1]"
  Water Column25 : TransferFcn  Numerator="[-CAN_T_W  1]"  Denominator="[0.5*CAN_T_W  1]"
  Water Column26 : TransferFcn  Numerator="[-WIM_T_W  1]"  Denominator="[0.5*WIM_T_W  1]"
  Water Column27 : TransferFcn  Numerator="[-WIM_T_W  1]"  Denominator="[0.5*WIM_T_W  1]"
  Water Column28 : TransferFcn  Numerator="[-VIC_T_W  1]"  Denominator="[0.5*VIC_T_W  1]"
  Water Column29 : TransferFcn  Numerator="[-VIC_T_W  1]"  Denominator="[0.5*VIC_T_W  1]"
  Water Column3 : TransferFcn  Numerator="[-RAN_T_W  1]"  Denominator="[0.5 * RAN_T_W   1]"
  Water Column30 : TransferFcn  Numerator="[-VIC_T_W  1]"  Denominator="[0.5*VIC_T_W  1]"
  Water Column31 : TransferFcn  Numerator="[-KOT_T_W  1]"  Denominator="[0.5*KOT_T_W  1]"
  Water Column32 : TransferFcn  Numerator="[-KOT_T_W  1]"  Denominator="[0.5*KOT_T_W  1]"
  Water Column33 : TransferFcn  Numerator="[-UKT_T_W  1]"  Denominator="[0.5*UKT_T_W  1]"
  Water Column34 : TransferFcn  Numerator="[-UKT_T_W  1]"  Denominator="[0.5*UKT_T_W  1]"
  Water Column35 : TransferFcn  Numerator="[-KOT_T_W  1]"  Denominator="[0.5*KOT_T_W  1]"
  Water Column4 : TransferFcn  Numerator="[-RTB_T_W  1]"  Denominator="[0.5 * RTB_T_W   1]"
  Water Column5 : TransferFcn  Numerator="[-RTB_T_W  1]"  Denominator="[0.5 * RTB_T_W   1]"
  Water Column6 : TransferFcn  Numerator="[-BWT_T_W  1]"  Denominator="[0.5 * BWT_T_W   1]"
  Water Column7 : TransferFcn  Numerator="[-UKU_T_W  1]"  Denominator="[0.5 * UKU_T_W   1]"
  Water Column8 : TransferFcn  Numerator="[-UKU_T_W  1]"  Denominator="[0.5 * UKU_T_W   1]"
  Water Column9 : TransferFcn  Numerator="[-NLX_T_W  1]"  Denominator="[0.5*NLX_T_W  1]"
  | Gain: F_GT : Gain  Gain=KEL_CC_F_GT
  Frequency Response : Outport
  wires:
  Governer 1/1 -> Turbine Dynamics (Reheat)/1
  Turbine Dynamics (Reheat)/1 -> Scaling 1/1
  Sum/1 -> Scope2/1, Frequency Response/1
  Constant/1 -> Sum/1
  Scaling 1/1 -> Add/1
  Governer 2/1 -> Turbine Dynamics (Reheat)1/1
  Turbine Dynamics (Reheat)1/1 -> Scaling 2/1
  Scaling 2/1 -> Add/2
  Governer/1 -> Turbine Dynamics (Reheat)2/1
  Turbine Dynamics (Reheat)2/1 -> Scaling 3/1
  Scaling 3/1 -> Add/3
  Add/1 -> Gain/1, Scope3/1, [LAK]
  [P_acc] -> " "/1
  " "/1 -> [Rotor_Dev]
  [Rotor_Dev] -> Gain3/1
  [LAK] -> Add1/2
  Load Disturbance/1 -> Add1/1
  Switch1/1 -> PURE DROOP4/1, PURE DROOP3/1
  Base Scaling Gain/1 -> Add2/1
  Add2/1 -> Gain18/1, Scope1/1, [SAM]
  Transient Droop/1 -> Water Column/1
  Water Column/1 -> Base Scaling Gain/1
  Water Column1/1 -> Base Scaling Gain1/1
  Transient Droop1/1 -> Water Column1/1
  Base Scaling Gain1/1 -> Add2/2
  [SAM] -> Add1/3
  Gain3/1 -> Sum/2
  Switch2/1 -> PURE DROOP8/1, PURE DROOP7/1, PURE DROOP6/1, PURE DROOP11/1, PURE DROOP10/1, PURE DROOP9/1
  Governer 7/1 -> Governer 8/1
  Governer 8/1 -> Base Scaling Gain3/1
  Governer 9/1 -> Governer 10/1
  Governer 10/1 -> Base Scaling Gain4/1
  Governer 11/1 -> Governer 12/1
  Governer 12/1 -> Base Scaling Gain5/1
  Governer 13/1 -> Governer 14/1
  Governer 14/1 -> Base Scaling Gain6/1
  Governer 15/1 -> Governer 16/1
  Governer 16/1 -> Base Scaling Gain7/1
  Governer 17/1 -> Combustr/1
  HRSG Delay/1 -> Gain1/1
  Combustr/1 -> HRSG Delay/1, | Gain: F_GT/1
  | Gain: F_GT/1 -> Scaling/1
  Gain1/1 -> Scaling/3
  Scaling/1 -> Gain2/1
  Base Scaling Gain3/1 -> Add3/1
  Base Scaling Gain4/1 -> Add3/2
  Base Scaling Gain5/1 -> Add3/3
  Base Scaling Gain6/1 -> Add3/4
  Base Scaling Gain7/1 -> Add3/5
  Gain2/1 -> Add3/6
  Add3/1 -> Gain4/1, Scope9/1, [KEL]
  [KEL] -> Add1/4
  Actuator Delay2/1 -> Scaling 6/1
  Add4/1 -> Scope4/1, [UTH]
  Scaling 6/1 -> Add4/3
  Governer 19/1 -> Actuator Delay1/1
  Governer1/1 -> Actuator Delay2/1
  Scaling 4/1 -> Add4/1
  Switch3/1 -> PURE DROOP14/1, PURE DROOP13/1, PURE DROOP12/1
  Actuator Delay1/1 -> Scaling 5/1
  Governer 18/1 -> Actuator Delay/1
  Scaling 5/1 -> Add4/2
  Actuator Delay/1 -> Scaling 4/1
  [UTH] -> Add1/5
  Switch4/1 -> PURE DROOP15/1, PURE DROOP16/1
  Transient Droop2/1 -> Water Column2/1
  Base Scaling Gain8/1 -> Add5/1
  Water Column2/1 -> Base Scaling Gain8/1
  Transient Droop3/1 -> Water Column3/1
  Water Column3/1 -> Base Scaling Gain9/1
  Base Scaling Gain9/1 -> Add5/2
  [RAN] -> Add1/6
  Switch5/1 -> PURE DROOP17/1, PURE DROOP5/1
  Water Column4/1 -> Base Scaling Gain2/1
  Base Scaling Gain2/1 -> Add6/1
  Base Scaling Gain10/1 -> Add6/2
  Transient Droop4/1 -> Water Column4/1
  [RTB] -> Add1/7
  Transient Droop5/1 -> Water Column5/1
  Water Column5/1 -> Base Scaling Gain10/1
  Transient Droop6/1 -> Water Column6/1
  Switch6/1 -> PURE DROOP19/1
  Water Column6/1 -> Base Scaling Gain12/1
  Base Scaling Gain12/1 -> Scope7/1, [BWT]
  [BWT] -> Add1/8
  Transient Droop7/1 -> Water Column7/1
  Base Scaling Gain13/1 -> Add7/1
  Switch7/1 -> PURE DROOP18/1, PURE DROOP20/1
  Water Column7/1 -> Base Scaling Gain13/1
  Add7/1 -> Scope8/1, [UKU]
  Base Scaling Gain11/1 -> Add7/2
  Water Column8/1 -> Base Scaling Gain11/1
  Transient Droop8/1 -> Water Column8/1
  [UKU] -> Add1/9
  [MAN] -> Add1/10
  Water Column10/1 -> Base Scaling Gain18/1
  Water Column11/1 -> Base Scaling Gain19/1
  Governer 6/1 -> Transient Droop10/1
  Base Scaling Gain GT2/1 -> Add9/1
  Base Scaling Gain17/1 -> Add10/1
  Transient Droop10/1 -> Water Column10/1
  Governer GT2/1 -> Transient Droop GT2/1
  Transient Droop9/1 -> Water Column9/1
  Base Scaling Gain GT/1 -> Add8/1
  Base Scaling Gain15/1 -> Add9/2
  Governer ST/1 -> Transient Droop ST/1
  Transient Droop GT/1 -> Base Scaling Gain GT/1
  Switch9/1 -> PURE DROOP GT1/1, PURE DROOP GT/1, PURE DROOP ST/1
  Base Scaling Gain GT1/1 -> Add8/2
  Transient Droop GT1/1 -> Base Scaling Gain GT1/1
  Governer 3/1 -> Transient Droop11/1
  Switch11/1 -> PURE DROOP25/1, PURE DROOP24/1
  Governer 5/1 -> Transient Droop9/1
  Base Scaling Gain19/1 -> Add11/1
  Base Scaling Gain18/1 -> Add10/2
  Transient Droop GT2/1 -> Base Scaling Gain GT2/1
  Governer GT/1 -> Transient Droop GT/1
  Transient Droop ST/1 -> Base Scaling Gain16/1
  Governer 4/1 -> Transient Droop12/1
  Switch8/1 -> PURE DROOP23/1, PURE DROOP22/1
  Switch10/1 -> PURE DROOP ST1/1, PURE DROOP GT2/1
  Add11/1 -> Scope14/1, [POL]
  Base Scaling Gain20/1 -> Add11/2
  Transient Droop ST1/1 -> Base Scaling Gain15/1
  Transient Droop11/1 -> Water Column11/1
  Governer GT1/1 -> Transient Droop GT1/1
  Base Scaling Gain16/1 -> Add8/3
  Water Column9/1 -> Base Scaling Gain17/1
  Water Column12/1 -> Base Scaling Gain20/1
  Governer ST1/1 -> Transient Droop ST1/1
  Transient Droop12/1 -> Water Column12/1
  [NLX] -> Add1/13
  [YUGA] -> Add1/12
  [SOBA] -> Add1/11
  [POL] -> Add1/14
  Base Scaling Gain33/1 -> Add16/2
  Transient Droop21/1 -> Water Column21/1
  Add14/1 -> Scope18/1, [OLX]
  Governer 29/1 -> Transient Droop19/1
  Switch17/1 -> PURE DROOP39/1, PURE DROOP38/1
  Base Scaling Gain21/1 -> Add18/1
  Governer 27/1 -> Transient Droop18/1
  Base Scaling Gain24/1 -> Add19/2
  Governer 33/1 -> Transient Droop23/1
  Base Scaling Gain32/1 -> Add16/1
  Transient Droop20/1 -> Water Column20/1
  Water Column15/1 -> Base Scaling Gain25/1
  Water Column23/1 -> Base Scaling Gain33/1
  Base Scaling Gain31/1 -> Add15/2
  Governer 26/1 -> Transient Droop15/1
  Base Scaling Gain30/1 -> Add15/1
  Water Column21/1 -> Base Scaling Gain31/1
  Base Scaling Gain28/1 -> Add13/2
  Governer 30/1 -> Transient Droop20/1
  Switch15/1 -> PURE DROOP31/1, PURE DROOP32/1
  Water Column13/1 -> Base Scaling Gain23/1
  Governer 28/1 -> Transient Droop17/1
  Switch12/1 -> PURE DROOP26/1, PURE DROOP40/1
  Switch14/1 -> PURE DROOP29/1, PURE DROOP30/1
  Transient Droop19/1 -> Water Column19/1
  Add18/1 -> Scope22/1, [WIM]
  Water Column18/1 -> Base Scaling Gain28/1
  Add13/1 -> Add14/2, Scope17/1
  Water Column22/1 -> Base Scaling Gain32/1
  Transient Droop14/1 -> Water Column14/1
  Governer 24/1 -> Transient Droop13/1
  Transient Droop15/1 -> Water Column15/1
  Base Scaling Gain27/1 -> Add13/1
  Switch23/1 -> PURE DROOP35/1, PURE DROOP33/1, PURE DROOP34/1
  Water Column24/1 -> Base Scaling Gain34/1
  Transient Droop22/1 -> Water Column22/1
  Water Column16/1 -> Base Scaling Gain26/1
  Transient Droop18/1 -> Water Column18/1
  Governer 25/1 -> Transient Droop16/1
  Transient Droop17/1 -> Water Column17/1
  Water Column14/1 -> Base Scaling Gain24/1
  Base Scaling Gain22/1 -> Add18/2
  Switch13/1 -> PURE DROOP27/1, PURE DROOP28/1
  Governer 21/1 -> Transient Droop27/1
  Transient Droop16/1 -> Water Column16/1
  Base Scaling Gain29/1 -> Add13/3
  Transient Droop26/1 -> Water Column26/1
  Governer 23/1 -> Transient Droop14/1
  Transient Droop27/1 -> Water Column27/1
  Switch16/1 -> PURE DROOP37/1, PURE DROOP36/1
  Base Scaling Gain23/1 -> Add19/1
  Transient Droop13/1 -> Water Column13/1
  Water Column25/1 -> Base Scaling Gain35/1
  Governer 20/1 -> Transient Droop25/1
  Add19/1 -> Scope15/1, [BRO]
  Transient Droop25/1 -> Water Column25/1
  Water Column17/1 -> Base Scaling Gain27/1
  Base Scaling Gain34/1 -> Add17/1
  Governer 34/1 -> Transient Droop24/1
  Transient Droop24/1 -> Water Column24/1
  Governer 22/1 -> Transient Droop26/1
  Base Scaling Gain26/1 -> Add12/2
  Add16/1 -> Scope20/1, [KUK]
  Base Scaling Gain35/1 -> Add17/2
  Water Column26/1 -> Base Scaling Gain21/1
  Add17/1 -> Scope21/1, [CAN]
  Add12/1 -> Add14/1, Scope16/1
  Governer 32/1 -> Transient Droop22/1
  Governer 31/1 -> Transient Droop21/1
  Water Column27/1 -> Base Scaling Gain22/1
  Water Column20/1 -> Base Scaling Gain30/1
  Transient Droop23/1 -> Water Column23/1
  Water Column19/1 -> Base Scaling Gain29/1
  Base Scaling Gain25/1 -> Add12/1
  [BRO] -> Add1/17
  [WIM] -> Add1/16
  [UMA] -> Add1/19
  [CAN] -> Add1/15
  [KUK] -> Add1/20
  [OLX] -> Add1/18
  Scaling 22/1 -> Add26/4
  Governer13/1 -> Actuator Delay17/1
  Base Scaling Gain37/1 -> Add20/2
  Actuator Delay5/1 -> Scaling 15/1
  Actuator Delay15/1 -> Scaling 16/1
  Actuator Delay14/1 -> Scaling 19/1
  Switch18/1 -> PURE DROOP41/1, PURE DROOP42/1, PURE DROOP43/1
  Governer 35/1 -> Transient Droop28/1
  Scaling 20/1 -> Add26/1
  Scaling 14/1 -> Add24/3
  Water Column33/1 -> Base Scaling Gain41/1
  Water Column32/1 -> Base Scaling Gain40/1
  Scaling 18/1 -> Add24/6
  Scaling 11/1 -> Add24/1
  Water Column30/1 -> Base Scaling Gain38/1
  Actuator Delay10/1 -> Scaling 17/1
  Actuator Delay7/1 -> Scaling 12/1
  Actuator Delay8/1 -> Scaling 13/1
  Scaling 7/1 -> Add23/1
  Scaling 19/1 -> Add26/2
  Actuator Delay4/1 -> Scaling 11/1
  Add22/1 -> Scope25/1, [UKT]
  Scaling 9/1 -> Add23/3
  Switch19/1 -> PURE DROOP48/1, PURE DROOP45/1, PURE DROOP44/1
  Actuator Delay11/1 -> Scaling 9/1
  Actuator Delay12/1 -> Scaling 8/1
  Actuator Delay13/1 -> Scaling 10/1
  Governer5/1 -> Actuator Delay5/1
  Base Scaling Gain40/1 -> Add21/2
  Governer3/1 -> Actuator Delay4/1
  Governer4/1 -> Actuator Delay13/1
  Governer10/1 -> Actuator Delay10/1
  Governer9/1 -> Actuator Delay9/1
  Governer6/1 -> Actuator Delay6/1
  Governer 43/1 -> Actuator Delay3/1
  Switch21/1 -> PURE DROOP49/1, PURE DROOP50/1, PURE DROOP51/1, PURE DROOP52/1, PURE DROOP60/1, PURE DROOP59/1, PURE DROOP58/1, PURE DROOP57/1, PURE DROOP56/1, PURE DROOP54/1, PURE DROOP53/1, PURE DROOP55/1
  Governer2/1 -> Actuator Delay11/1
  Scaling 8/1 -> Add23/2
  Add26/1 -> Scope26/1, [BAR]
  Actuator Delay3/1 -> Scaling 7/1
  Base Scaling Gain41/1 -> Add22/1
  Governer 44/1 -> Actuator Delay12/1
  Base Scaling Gain43/1 -> Add21/3
  Scaling 10/1 -> Add23/4
  Base Scaling Gain39/1 -> Add21/1
  Transient Droop32/1 -> Water Column32/1
  Water Column35/1 -> Base Scaling Gain43/1
  Governer 42/1 -> Transient Droop35/1
  Water Column31/1 -> Base Scaling Gain39/1
  Transient Droop35/1 -> Water Column35/1
  Transient Droop34/1 -> Water Column34/1
  Governer 39/1 -> Transient Droop32/1
  Governer 40/1 -> Transient Droop33/1
  Transient Droop31/1 -> Water Column31/1
  Water Column29/1 -> Base Scaling Gain37/1
  Governer 38/1 -> Transient Droop31/1
  Base Scaling Gain42/1 -> Add22/2
  Transient Droop29/1 -> Water Column29/1
  Governer7/1 -> Actuator Delay7/1
  Base Scaling Gain38/1 -> Add20/3
  Water Column28/1 -> Base Scaling Gain36/1
  Switch20/1 -> PURE DROOP47/1, PURE DROOP46/1
  Actuator Delay16/1 -> Scaling 21/1
  Actuator Delay17/1 -> Scaling 22/1
  Governer 46/1 -> Actuator Delay14/1
  Base Scaling Gain36/1 -> Add20/1
  Governer8/1 -> Actuator Delay8/1
  Scaling 13/1 -> Add24/5
  Governer11/1 -> Actuator Delay15/1
  Governer 45/1 -> Actuator Delay18/1
  Transient Droop30/1 -> Water Column30/1
  Scaling 17/1 -> Add24/7
  Actuator Delay18/1 -> Scaling 20/1
  Governer12/1 -> Actuator Delay16/1
  Transient Droop33/1 -> Water Column33/1
  Governer 36/1 -> Transient Droop29/1
  Scaling 12/1 -> Add24/4
  Add23/1 -> Add25/1
  Governer 41/1 -> Transient Droop34/1
  Scaling 16/1 -> Add24/8
  Scaling 15/1 -> Add24/2
  Actuator Delay9/1 -> Scaling 18/1
  Transient Droop28/1 -> Water Column28/1
  Scaling 21/1 -> Add26/3
  Actuator Delay6/1 -> Scaling 14/1
  Governer 37/1 -> Transient Droop30/1
  Water Column34/1 -> Base Scaling Gain42/1
  Add24/1 -> Add25/2
  [VIC] -> Add1/21
  [UKT] -> Add1/23
  [SAP] -> Add1/24
  [BAR] -> Add1/25
  [KOT] -> Add1/22
  PURE DROOP/1 -> Add27/2
  Add27/1 -> Governer 1/1
  [MAD] -> Add1/26
  [LAU] -> Add1/27
  Inverter Delay4/1 -> Base Scaling Gain47/1
  [UPP] -> Add1/29
  Constant1/1 -> Add27/1
  Constant2/1 -> Governer 47/1
  Governer 47/1 -> Scope32/1
  Add29/1 -> Transient Droop/1
  PURE DROOP3/1 -> Add29/2
  Constant4/1 -> Add29/1
  Add30/1 -> Governer 7/1
  PURE DROOP6/1 -> Add30/2
  Constant5/1 -> Add30/1
  Constant14/1 -> Inverter Delay4/1
  Inverter Delay1/1 -> Base Scaling Gain44/1
  Base Scaling Gain44/1 -> Gain13/1, Scope28/1, Add28/1, [MAD]
  Constant11/1 -> Inverter Delay1/1
  Constant12/1 -> Inverter Delay2/1
  Inverter Delay2/1 -> Base Scaling Gain45/1
  Constant13/1 -> Inverter Delay3/1
  Inverter Delay3/1 -> Base Scaling Gain46/1
  Add28/1 -> [SOL_TOTAL]
  [SOL_TOTAL] -> To Workspace/1
  PURE DROOP1/1 -> Add35/2
  Add35/1 -> Governer 2/1
  Constant15/1 -> Add35/1
  PURE DROOP2/1 -> Add36/2
  Add36/1 -> Governer/1
  Constant16/1 -> Add36/1
  PURE DROOP4/1 -> Add37/2
  Add37/1 -> Transient Droop1/1
  Constant17/1 -> Add37/1
  Constant18/1 -> Add38/1
  PURE DROOP7/1 -> Add38/2
  Add38/1 -> Governer 9/1
  Constant19/1 -> Add39/1
  PURE DROOP8/1 -> Add39/2
  Add39/1 -> Governer 11/1
  Constant20/1 -> Add40/1
  Add40/1 -> Governer 13/1
  PURE DROOP9/1 -> Add40/2
  PURE DROOP10/1 -> Add41/2
  Add41/1 -> Governer 15/1
  Constant21/1 -> Add41/1
  Constant22/1 -> Add42/1
  PURE DROOP11/1 -> Add42/2
  Add42/1 -> Governer 17/1
  Add43/1 -> Governer 5/1
  Constant23/1 -> Add43/1
  PURE DROOP22/1 -> Add43/2
  Add44/1 -> Governer 6/1
  Constant24/1 -> Add44/1
  PURE DROOP23/1 -> Add44/2
  Constant25/1 -> Add45/1
  PURE DROOP36/1 -> Add45/2
  Add45/1 -> Governer 30/1
  PURE DROOP37/1 -> Add46/2
  Constant26/1 -> Add46/1
  Add46/1 -> Governer 31/1
  PURE DROOP41/1 -> Add47/2
  Constant27/1 -> Add47/1
  Add47/1 -> Governer 35/1
  Constant28/1 -> Add48/1
  Add48/1 -> Governer 36/1
  PURE DROOP42/1 -> Add48/2
  Constant29/1 -> Add49/1
  Add49/1 -> Governer 37/1
  PURE DROOP43/1 -> Add49/2
  Constant30/1 -> Add50/1
  Add50/1 -> Governer 38/1
  PURE DROOP44/1 -> Add50/2
  Constant31/1 -> Add51/1
  PURE DROOP45/1 -> Add51/2
  Add51/1 -> Governer 39/1
  Constant32/1 -> Add52/1
  PURE DROOP48/1 -> Add52/2
  Add52/1 -> Governer 42/1
  PURE DROOP GT/1 -> Add31/2
  Add31/1 -> Governer GT/1
  Constant6/1 -> Add31/1
  Add32/1 -> Governer GT1/1
  PURE DROOP GT1/1 -> Add32/2
  Constant7/1 -> Add32/1
  Add33/1 -> Governer ST/1
  PURE DROOP ST/1 -> Add33/2
  Constant8/1 -> Add33/1
  PURE DROOP49/1 -> Add34/2
  Add34/1 -> Governer 43/1
  Constant33/1 -> Add34/1
  Constant34/1 -> Add53/1
  Add53/1 -> Governer 44/1
  PURE DROOP50/1 -> Add53/2
  Constant35/1 -> Add54/1
  Add54/1 -> Governer2/1
  PURE DROOP51/1 -> Add54/2
  Constant36/1 -> Add55/1
  Add55/1 -> Governer4/1
  PURE DROOP52/1 -> Add55/2
  Constant37/1 -> Add56/1
  Add56/1 -> Governer3/1
  PURE DROOP55/1 -> Add56/2
  Add57/1 -> Governer5/1
  Constant38/1 -> Add57/1
  PURE DROOP53/1 -> Add57/2
  Add58/1 -> Governer6/1
  Constant39/1 -> Add58/1
  PURE DROOP54/1 -> Add58/2
  Add59/1 -> Governer7/1
  Constant40/1 -> Add59/1
  PURE DROOP56/1 -> Add59/2
  Add60/1 -> Governer8/1
  Constant41/1 -> Add60/1
  PURE DROOP57/1 -> Add60/2
  Add61/1 -> Governer9/1
  Constant42/1 -> Add61/1
  PURE DROOP58/1 -> Add61/2
  Add62/1 -> Governer10/1
  Constant43/1 -> Add62/1
  PURE DROOP59/1 -> Add62/2
  Add63/1 -> Governer11/1
  Constant44/1 -> Add63/1
  PURE DROOP60/1 -> Add63/2
  Constant45/1 -> Add64/1
  PURE DROOP GT2/1 -> Add64/2
  Add64/1 -> Governer GT2/1
  PURE DROOP ST1/1 -> Add65/2
  Add65/1 -> Governer ST1/1
  Constant46/1 -> Add65/1
  Constant9/1 -> Scaling/2
  Inverter Delay/1 -> Base Scaling Gain14/1
  Constant10/1 -> Inverter Delay/1
  Base Scaling Gain49/1 -> Add28/4, [HBT]
  Inverter Delay5/1 -> Base Scaling Gain49/1
  Constant47/1 -> Inverter Delay5/1
  Constant48/1 -> Inverter Delay6/1
  Base Scaling Gain50/1 -> Add28/5, [SAG]
  Inverter Delay6/1 -> Base Scaling Gain50/1
  Constant49/1 -> Inverter Delay7/1
  Base Scaling Gain51/1 -> Add28/6, [SS1]
  Inverter Delay7/1 -> Base Scaling Gain51/1
  Constant50/1 -> Inverter Delay8/1
  Base Scaling Gain52/1 -> Add28/7, [SS2]
  Inverter Delay8/1 -> Base Scaling Gain52/1
  [HBT] -> Add1/30
  [SAG] -> Add1/31
  [SS1] -> Add1/32
  [SS2] -> Add1/33
  Constant51/1 -> Inverter Delay9/1
  Base Scaling Gain53/1 -> Scope33/1, Add66/3, [AMB]
  Inverter Delay9/1 -> Base Scaling Gain53/1
  Constant52/1 -> Inverter Delay10/1
  Base Scaling Gain54/1 -> Add66/4, Scope34/1, [MADU]
  Inverter Delay10/1 -> Base Scaling Gain54/1
  Constant53/1 -> Inverter Delay11/1
  Base Scaling Gain55/1 -> Scope35/1, Add66/5, [MAM1]
  Inverter Delay11/1 -> Base Scaling Gain55/1
  Constant54/1 -> Inverter Delay12/1
  Base Scaling Gain56/1 -> Scope36/1, Add66/6, [MAM2]
  Inverter Delay12/1 -> Base Scaling Gain56/1
  Constant55/1 -> Inverter Delay13/1
  Base Scaling Gain57/1 -> Scope37/1, Add66/7, [MAM3]
  Inverter Delay13/1 -> Base Scaling Gain57/1
  Constant56/1 -> Inverter Delay14/1
  Base Scaling Gain58/1 -> Scope38/1, Add66/8, [NAL]
  Inverter Delay14/1 -> Base Scaling Gain58/1
  Constant57/1 -> Inverter Delay15/1
  Base Scaling Gain59/1 -> Scope39/1, Add66/9, [NIR]
  Inverter Delay15/1 -> Base Scaling Gain59/1
  Constant58/1 -> Inverter Delay16/1
  Base Scaling Gain60/1 -> Scope40/1, Add66/10, [PWD]
  Inverter Delay16/1 -> Base Scaling Gain60/1
  Constant59/1 -> Inverter Delay17/1
  Base Scaling Gain61/1 -> Scope41/1, Add66/11, [POLW]
  Inverter Delay17/1 -> Base Scaling Gain61/1
  Constant60/1 -> Inverter Delay18/1
  Base Scaling Gain62/1 -> Scope42/1, Add66/12, [SEG]
  Inverter Delay18/1 -> Base Scaling Gain62/1
  Constant62/1 -> Inverter Delay20/1
  Base Scaling Gain64/1 -> Scope44/1, Add66/13, [VALL]
  Inverter Delay20/1 -> Base Scaling Gain64/1
  Constant63/1 -> Inverter Delay21/1
  Base Scaling Gain65/1 -> Scope45/1, Add66/14, [VID]
  Inverter Delay21/1 -> Base Scaling Gain65/1
  Constant64/1 -> Inverter Delay22/1
  Base Scaling Gain66/1 -> Scope46/1, Add66/15, [WILL]
  Inverter Delay22/1 -> Base Scaling Gain66/1
  Constant65/1 -> Inverter Delay23/1
  Base Scaling Gain67/1 -> Scope47/1, Add66/16, [WSC]
  Inverter Delay23/1 -> Base Scaling Gain67/1
  Add66/1 -> [WIND_TOT]
  [WIND_TOT] -> To Workspace1/1
  [AMB] -> Add1/34
  [MADU] -> Add1/35
  [MAM1] -> Add1/36
  [MAM2] -> Add1/37
  [MAM3] -> Add1/38
  [NAL] -> Add1/39
  [NIR] -> Add1/40
  [PWD] -> Add1/41
  [POLW] -> Add1/42
  [SEG] -> Add1/43
  [VALL] -> Add1/44
  [VID] -> Add1/45
  [WILL] -> Add1/46
  [SOC] -> Add1/28
  [WSC] -> Add1/47
  Gain/1 -> Display/1
  Gain18/1 -> Display1/1
  Gain4/1 -> Display2/1
  Add5/1 -> Scope5/1, [RAN]
  Add6/1 -> Scope6/1, [RTB]
  Add10/1 -> Gain5/1, Scope13/1, [NLX]
  Gain5/1 -> Display4/1
  Gain6/1 -> Display3/1
  Add8/1 -> Gain6/1, Scope11/1, [YUGA]
  Add9/1 -> Gain7/1, Scope12/1, [SOBA]
  Gain7/1 -> Display5/1
  Add15/1 -> Gain9/1, Scope19/1, [UMA]
  Gain9/1 -> Display6/1
  Add20/1 -> Gain10/1, Scope23/1, [VIC]
  Gain10/1 -> Display7/1
  Add21/1 -> Gain11/1, Scope24/1, [KOT]
  Gain11/1 -> Display8/1
  Gain12/1 -> Display9/1
  Add25/1 -> Gain12/1, Scope27/1, [SAP]
  Gain13/1 -> Display10/1
  Base Scaling Gain45/1 -> Gain14/1, Scope29/1, Add28/2, [LAU]
  Gain14/1 -> Display11/1
  Base Scaling Gain46/1 -> Gain15/1, Scope30/1, Add28/3, [SOC]
  Gain15/1 -> Display12/1
  Base Scaling Gain14/1 -> Gain16/1, Scope10/1, Add66/2, [MAN]
  Gain16/1 -> Display13/1
  PURE DROOP12/1 -> Add67/2
  PURE DROOP13/1 -> Add68/2
  PURE DROOP14/1 -> Add69/2
  Add67/1 -> Governer 18/1
  Add68/1 -> Governer 19/1
  Add69/1 -> Governer1/1
  Constant61/1 -> Add67/1
  Constant66/1 -> Add68/1
  Constant67/1 -> Add69/1
  Add71/1 -> Transient Droop3/1
  Add70/1 -> Transient Droop2/1
  PURE DROOP15/1 -> Add70/2
  PURE DROOP16/1 -> Add71/2
  Constant69/1 -> Add71/1
  Constant68/1 -> Add70/1
  Add72/1 -> Transient Droop4/1
  Add73/1 -> Transient Droop5/1
  PURE DROOP5/1 -> Add72/2
  PURE DROOP17/1 -> Add73/2
  Constant70/1 -> Add72/1
  Constant71/1 -> Add73/1
  Add74/1 -> Transient Droop6/1
  PURE DROOP19/1 -> Add74/2
  Constant72/1 -> Add74/1
  Add75/1 -> Transient Droop7/1
  Add76/1 -> Transient Droop8/1
  Constant73/1 -> Add75/1
  Constant74/1 -> Add76/1
  PURE DROOP20/1 -> Add75/2
  PURE DROOP18/1 -> Add76/2
  Add77/1 -> Governer 3/1
  Add78/1 -> Governer 4/1
  PURE DROOP24/1 -> Add77/2
  PURE DROOP25/1 -> Add78/2
  Constant75/1 -> Add78/1
  Constant76/1 -> Add77/1
  Add80/1 -> Governer 34/1
  Add79/1 -> Governer 20/1
  PURE DROOP40/1 -> Add80/2
  PURE DROOP26/1 -> Add79/2
  Constant77/1 -> Add80/1
  Constant78/1 -> Add79/1
  Add82/1 -> Governer 21/1
  Add81/1 -> Governer 22/1
  Constant79/1 -> Add81/1
  Constant80/1 -> Add82/1
  PURE DROOP28/1 -> Add81/2
  PURE DROOP27/1 -> Add82/2
  Add84/1 -> Governer 24/1
  Add83/1 -> Governer 23/1
  PURE DROOP30/1 -> Add84/2
  PURE DROOP29/1 -> Add83/2
  Constant81/1 -> Add84/1
  Constant82/1 -> Add83/1
  Add85/1 -> Governer 26/1
  Add86/1 -> Governer 25/1
  Add87/1 -> Governer 28/1
  Add88/1 -> Governer 27/1
  PURE DROOP32/1 -> Add85/2
  PURE DROOP31/1 -> Add86/2
  PURE DROOP34/1 -> Add87/2
  PURE DROOP33/1 -> Add88/2
  PURE DROOP35/1 -> Add89/2
  Add89/1 -> Governer 29/1
  Constant84/1 -> Add86/1
  Constant83/1 -> Add85/1
  Constant85/1 -> Add87/1
  Constant86/1 -> Add88/1
  Constant87/1 -> Add89/1
  Add91/1 -> Governer 33/1
  PURE DROOP39/1 -> Add91/2
  Add90/1 -> Governer 32/1
  PURE DROOP38/1 -> Add90/2
  Constant89/1 -> Add91/1
  Constant88/1 -> Add90/1
  Add93/1 -> Governer 41/1
  Add92/1 -> Governer 40/1
  PURE DROOP46/1 -> Add92/2
  PURE DROOP47/1 -> Add93/2
  Constant91/1 -> Add93/1
  Constant90/1 -> Add92/1
  Add97/1 -> Governer13/1
  Add96/1 -> Governer12/1
  Add95/1 -> Governer 46/1
  Add94/1 -> Governer 45/1
  PURE DROOP61/1 -> Add94/2
  PURE DROOP62/1 -> Add95/2
  PURE DROOP63/1 -> Add96/2
  PURE DROOP64/1 -> Add97/2
  Constant92/1 -> Add94/1
  Constant93/1 -> Add95/1
  Constant94/1 -> Add96/1
  Constant95/1 -> Add97/1
  [Rotor_Dev] -> "Switch "/1
  Constant96/1 -> "Switch "/3
  [Rotor_Dev] -> Switch1/1
  Constant97/1 -> Switch1/3
  [Rotor_Dev] -> Switch2/1
  Constant98/1 -> Switch2/3
  [Rotor_Dev] -> Switch3/1
  Constant99/1 -> Switch3/3
  [Rotor_Dev] -> Switch4/1
  Constant100/1 -> Switch4/3
  [Rotor_Dev] -> Switch5/1
  Constant101/1 -> Switch5/3
  [Rotor_Dev] -> Switch6/1
  Constant102/1 -> Switch6/3
  [Rotor_Dev] -> Switch7/1
  Constant103/1 -> Switch7/3
  [Rotor_Dev] -> Switch8/1
  Constant104/1 -> Switch8/3
  [Rotor_Dev] -> Switch9/1
  Constant105/1 -> Switch9/3
  [Rotor_Dev] -> Switch10/1
  Constant106/1 -> Switch10/3
  [Rotor_Dev] -> Switch11/1
  Constant107/1 -> Switch11/3
  [Rotor_Dev] -> Switch12/1
  Constant108/1 -> Switch12/3
  [Rotor_Dev] -> Switch13/1
  Constant109/1 -> Switch13/3
  [Rotor_Dev] -> Switch14/1
  Constant110/1 -> Switch14/3
  [Rotor_Dev] -> Switch15/1
  Constant111/1 -> Switch15/3
  [Rotor_Dev] -> Switch16/1
  Constant112/1 -> Switch16/3
  [Rotor_Dev] -> Switch17/1
  Constant113/1 -> Switch17/3
  [Rotor_Dev] -> Switch18/1
  Constant114/1 -> Switch18/3
  [Rotor_Dev] -> Switch19/1
  Constant115/1 -> Switch19/3
  [Rotor_Dev] -> Switch20/1
  Constant116/1 -> Switch20/3
  [Rotor_Dev] -> Switch21/1
  Constant117/1 -> Switch21/3
  [Rotor_Dev] -> Switch22/1
  Constant118/1 -> Switch22/3
  Switch22/1 -> PURE DROOP64/1, PURE DROOP63/1, PURE DROOP61/1, PURE DROOP62/1
  Constant119/1 -> Switch22/2
  Constant120/1 -> Switch21/2
  Constant121/1 -> Switch20/2
  Constant122/1 -> Switch19/2
  Constant123/1 -> Switch18/2
  Constant124/1 -> Switch17/2
  Constant125/1 -> Switch16/2
  Constant126/1 -> Switch15/2
  Constant128/1 -> Switch23/2
  Constant127/1 -> Switch23/3
  [Rotor_Dev] -> Switch23/1
  Constant129/1 -> Switch14/2
  Constant130/1 -> Switch13/2
  Constant131/1 -> Switch12/2
  Constant132/1 -> Switch11/2
  Constant133/1 -> Switch10/2
  Constant134/1 -> Switch9/2
  Constant135/1 -> Switch8/2
  Constant136/1 -> Switch7/2
  Constant137/1 -> Switch6/2
  Constant138/1 -> Switch5/2
  Constant139/1 -> Switch4/2
  Constant140/1 -> Switch3/2
  Constant141/1 -> Switch2/2
  Constant142/1 -> Switch1/2
  "Switch "/1 -> PURE DROOP1/1, PURE DROOP/1, PURE DROOP2/1
  Constant143/1 -> "Switch "/2
  PURE DROOP21/1 -> Add98/2
  Constant146/1 -> Display15/1, Add98/1
  Transient Droop37/1 -> Base Scaling Gain63/1
  Constant144/1 -> Switch24/3
  Add98/1 -> Transient Droop37/1
  Constant145/1 -> Switch24/2
  Switch24/1 -> PURE DROOP21/1
  [Rotor_Dev] -> Switch24/1
  [AGG] -> Add1/48
  Gain17/1 -> Display14/1
  Base Scaling Gain63/1 -> Gain17/1, Scope43/1, [AGG]
  Add1/1 -> Scope/1, [P_acc]
  Gain8/1 -> Display16/1
  Base Scaling Gain47/1 -> Gain8/1, [UPP], Add66/1, Scope31/1
